simulink model "p_12"  (R2018b)
settings: Solver=VariableStepAuto  StartTime=0.0  StopTime=30  MaxStep=0.01  RelTol=1e-3
settings Model: Creator=kekos  LastModifiedBy=kekos

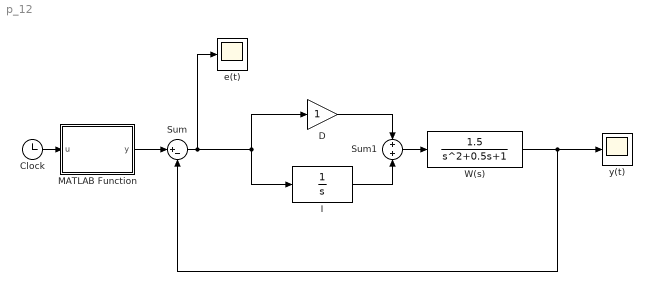
== system p_12 ==
  Clock : Clock
  D : Gain
  "I " : TransferFcn  Denominator=[1 0]
  MATLAB Function : MATLAB Function  TreatAsAtomicUnit=on
  Sum : Sum  Inputs=|+-
  Sum1 : Sum  Inputs=+|+
  W(s) : TransferFcn  Numerator=[1.5]  Denominator=[1 0.5 1]
  e(t) : Scope
  y(t) : Scope
  wires:
  Sum/1 -> D/1, "I "/1, e(t)/1
  W(s)/1 -> y(t)/1, Sum/2
  Clock/1 -> MATLAB Function/1(u)
  MATLAB Function/1(y) -> Sum/1
  "I "/1 -> Sum1/2
  Sum1/1 -> W(s)/1
  D/1 -> Sum1/1

== matlab function p_12/MATLAB Function ==
  data: u input; y output
function y = fcn(u)

y = 4*u;
